simulink model "check_model"  (R2021b)
settings: Solver=VariableStepAuto  StartTime=0.0  StopTime=100  FixedStep=0.1  RelTol=1e-3
libraries: slpidlib x1
settings Model: Creator=kairi  LastModifiedBy=kairi
settings RTWCC: GenCodeOnly=on

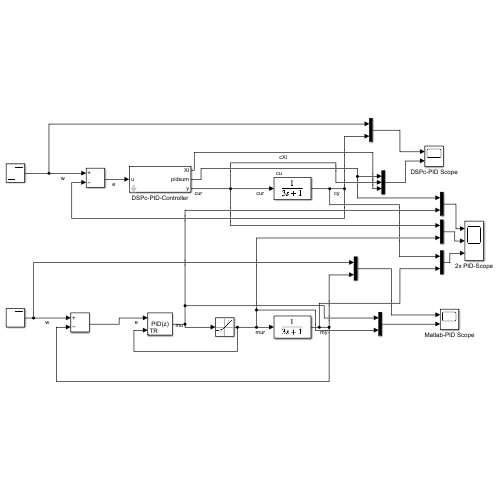
[thumbnail: Simulink's stored preview of the top-level diagram]
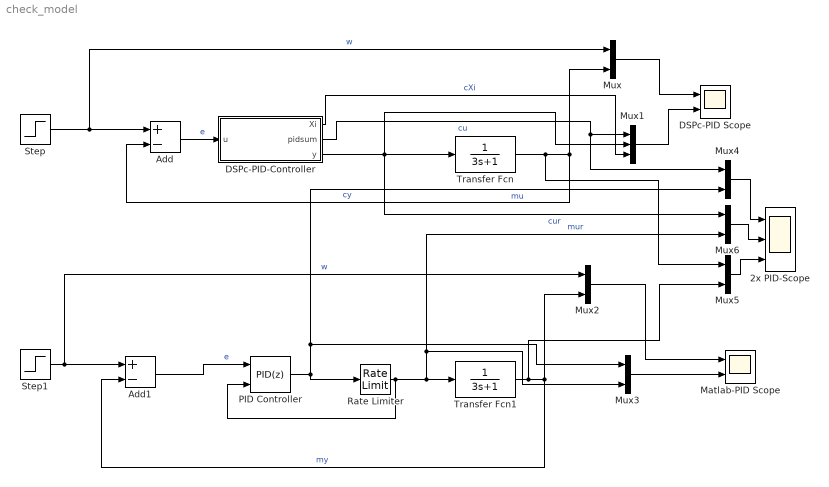
== system check_model ==
  2x PID-Scope : Scope  NumInputPorts=3
  Add : Sum  Inputs=+-
  Add1 : Sum  Inputs=+-
  DSPc-PID Scope : Scope  NumInputPorts=2
  DSPc-PID-Controller : Subsystem  mask{Kp=10, Ki=10 / 3, Kd=0, N=5, limit_output=off, upper_limit=1, lower_limit=0, limit_rate=on, rising_slew_rate=0.01, falling_slew_rate=-0.01, anti_windup_enabled=on, Kb=2/3, tracking_enabled=off, Kt=0}
      mask DialogControl Container3 Prompt: Controller
      mask DialogControl Container4 Prompt: Output
      mask DialogControl Container5 Prompt: Advanced
  Matlab-PID Scope : Scope  NumInputPorts=2
  Mux{,2..6} (6 alike) : Mux  Inputs=2
  Mux1 : Mux  Inputs=3
  PID Controller : slpidlib/PID Controller  Controller=PID  Form=Parallel  TimeDomain=Discrete-time  UseExternalTs=off  SampleTime=0.1  IntegratorMethod=Forward Euler  FilterMethod=Forward Euler  ControllerParametersSource=internal  P=1.47764760058376  I=0.927459772661165  D=-0.0909316657783639  UseFilter=on  N=5  TunerSelectOption=Transfer Function Based (PID Tuner App)  InitialConditionSource=internal  InitialConditionForIntegrator=0  InitialConditionForFilter=0  DifferentiatorICPrevScaledInput=0  ExternalReset=none  TrackingMode=on  Kt=2/3  LimitOutput=off  SatLimitsSource=internal  UpperSaturationLimit=inf  LowerSaturationLimit=-inf  LinearizeAsGain=on  AntiWindupMode=none  Kb=1  POutMin=[]  POutMax=[]  IOutMin=[]  IOutMax=[]  DOutMin=[]  DOutMax=[]  NOutMin=[]  NOutMax=[]  SumOutMin=[]  SumOutMax=[]  SaturationOutMin=[]  SaturationOutMax=[]  PParamMin=[]  PParamMax=[]  IParamMin=[]  IParamMax=[]  DParamMin=[]  DParamMax=[]  NParamMin=[]  NParamMax=[]  KbParamMin=[]  KbParamMax=[]  KtParamMin=[]  KtParamMax=[]  KbOutMin=[]  KbOutMax=[]  KtOutMin=[]  KtOutMax=[]  IntegratorOutMin=[]  IntegratorOutMax=[]  FilterOutMin=[]  FilterOutMax=[]  SumI1OutMin=[]  SumI1OutMax=[]  SumI2OutMin=[]  SumI2OutMax=[]  SumI3OutMin=[]  SumI3OutMax=[]  SumI4OutMin=[]  SumI4OutMax=[]  SumDOutMin=[]  SumDOutMax=[]  DifferentiatorOutMin=[]  DifferentiatorOutMax=[]  FilterDiffOutCoefMin=[]  FilterDiffOutCoefMax=[]  ReciprocalOutMin=[]  ReciprocalOutMax=[]  SumDenOutMin=[]  SumDenOutMax=[]  SumNumOutMin=[]  SumNumOutMax=[]  DivideOutMin=[]  DivideOutMax=[]  UdiffTsProdOutMin=[]  UdiffTsProdOutMax=[]  NTsProdOutMin=[]  NTsProdOutMax=[]  UintegralTsProdOutMin=[]  UintegralTsProdOutMax=[]  UngainTsProdOutMin=[]  UngainTsProdOutMax=[]  IntegratorContinuousStateAttributes=''  IntegratorStateMustResolveToSignalObject=off  IntegratorRTWStateStorageClass=Auto  FilterContinuousStateAttributes=''  FilterStateMustResolveToSignalObject=off  FilterRTWStateStorageClass=Auto  ParallelPVariant=InternalParameters  IdealPVariant=Disabled  IVariant=InternalParameters  DVariant=InternalParameters  IntegratorVariant=Discrete  SatVariant=Disabled  AWVariant=Passthrough  PCopyVariant=Disabled  TRVariant=Enabled  FdbkBlocksVariant=Forward  IdealPFdbkVariant=Disabled  SatFdbkVariant=Disabled  DerivativeFilterVariant=ForwardEulerFilter  NVariant=InternalParameters  NCopyVariant=Disabled  FilterICVariant=InternalICsFilter  IntegratorICVariant=InternalICs  ExternalResetVariant=Disabled  TRSumVariant=TrackingMode  SumFdbkVariant=Disabled  SumVariant=Sum_PID  TsampFilterVariant=InternalTs  TsampNgainVariant=Passthrough  TsampIntegralVariant=Passthrough  ExternalSaturationOutDataTypeStr=Inherit: Same as second input
  Rate Limiter : RateLimiter  RisingSlewLimit=0.01  FallingSlewLimit=-0.01  SampleTimeMode=inherited  LinearizeAsGain=off
  Step : Step  After=0.5  SampleTime=0
  Step1 : Step  After=0.5  SampleTime=0
  Transfer Fcn : TransferFcn  Denominator=[3 1]
  Transfer Fcn1 : TransferFcn  Denominator=[3 1]
  wires:
  Mux5/1 -> 2x PID-Scope/3
  Mux2/1 -> Matlab-PID Scope/1
  Mux6/1 -> 2x PID-Scope/2
  Mux3/1 -> Matlab-PID Scope/2
  Rate Limiter/1 -> PID Controller/2, Mux6/2, Mux3/2, Transfer Fcn1/1  "mur"
  Transfer Fcn/1 -> Mux5/1, Mux/2, Add/2  "cy"
  Mux/1 -> DSPc-PID Scope/1
  Mux4/1 -> 2x PID-Scope/1
  Add/1 -> DSPc-PID-Controller/1(u)  "e"
  PID Controller/1 -> Rate Limiter/1, Mux3/1, Mux4/2  "mu"
  Add1/1 -> PID Controller/1  "e"
  DSPc-PID-Controller/1(Xi) -> Mux1/3  "cXi"
  DSPc-PID-Controller/2(pidsum) -> Mux4/1, Mux1/1  "cu"
  Step1/1 -> Mux2/1, Add1/1  "w"
  Transfer Fcn1/1 -> Mux5/2, Mux2/2, Add1/2  "my"
  Mux1/1 -> DSPc-PID Scope/2
  DSPc-PID-Controller/3(y) -> Mux6/1, Mux1/2, Transfer Fcn/1  "cur"
  Step/1 -> Mux/1, Add/1  "w"

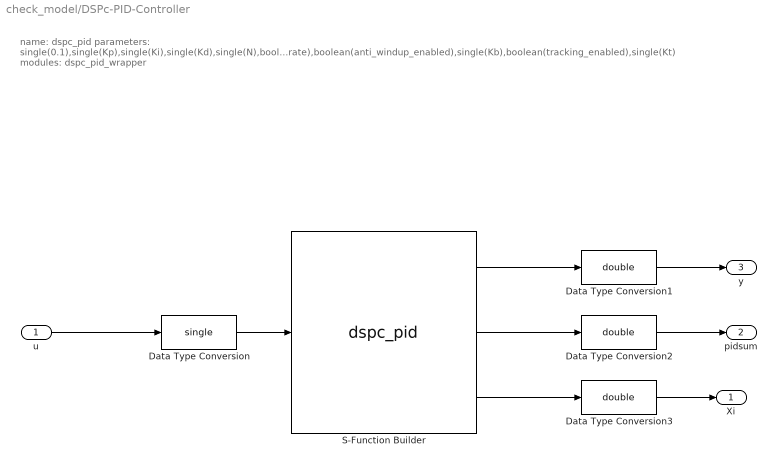
== system check_model/DSPc-PID-Controller ==
  note: name:
      | dspc_pid
      |
      | parameters:
      | single(0.1),single(Kp),single(Ki),single(Kd),single(N),boolean(limit_output),single(upper_limit),single(lower_limit),boolean(limit_rate),single(rising_slew_rate),single(falling_slew_rate),boolean(anti_windup_enabled),single(Kb),boolean(tracking_enabled),single(Kt)
      |
      | modules:
      | dspc_pid_wrapper
  u : Inport
  Data Type Conversion : DataTypeConversion  OutDataTypeStr=single
  Data Type Conversion1 : DataTypeConversion  OutDataTypeStr=double
  Data Type Conversion2 : DataTypeConversion  OutDataTypeStr=double
  Data Type Conversion3 : DataTypeConversion  OutDataTypeStr=double
  S-Function Builder : S-Function  FunctionName=dspc_pid  Parameters=single(0.1),single(Kp),single(Ki),single(Kd),single(N),boolean(limit_output),single(upper_limit),single(lower_limit),boolean(limit_rate),single(rising_slew_rate),single(falling_slew_rate),boolean(anti_windup_enabled),single(Kb),boolean(tracking_enabled),single(Kt)  SFunctionModules=dspc_pid_wrapper  SFunctionDeploymentMode=off  EnableBusSupport=off  mask(S-Function Builder){}
      mask help: Simulink:masks:SFunctionBuilder_MD
      mask init:
      | val = [[.9  0.75 0.75 1 1 .9 .9 1]',[1 1 0.75 0.75 .9 .9 1 .9]'];try , sys = get_param(gcb,'SfunBuilderFcnName');if isempty(sys), sys = get_param(gcb,'FunctionName'); end,catch, sys = get_param(gcb,'FunctionName'); end
      settings: CopyFcn=set_param(gcbh,'LinkStatus','none')  OpenFcn=sfunctionwizard(gcbh)
      mask Display:
      | plot(val(:,1),val(:,2))
      | disp(sys)
      | port_label('input',1,'u')
      | port_label('output',1,'y')
      | port_label('output',2,'pidsum')
      | port_label('output',3,'Xi')
  Xi : Outport
  pidsum : Outport  Port=2
  y : Outport  Port=3
  wires:
  u/1 -> Data Type Conversion/1
  S-Function Builder/1 -> Data Type Conversion1/1
  Data Type Conversion/1 -> S-Function Builder/1
  Data Type Conversion1/1 -> y/1
  S-Function Builder/2 -> Data Type Conversion2/1
  Data Type Conversion2/1 -> pidsum/1
  Data Type Conversion3/1 -> Xi/1
  S-Function Builder/3 -> Data Type Conversion3/1
